simulink subsystem "luces"  (R2023b)
settings: Solver=VariableStepAuto  StartTime=0.0  StopTime=10.0  RelTol=1e-3
libraries: simulink x8
settings Model: Creator=Usuario_UMA  LastModifiedBy=fdcdm

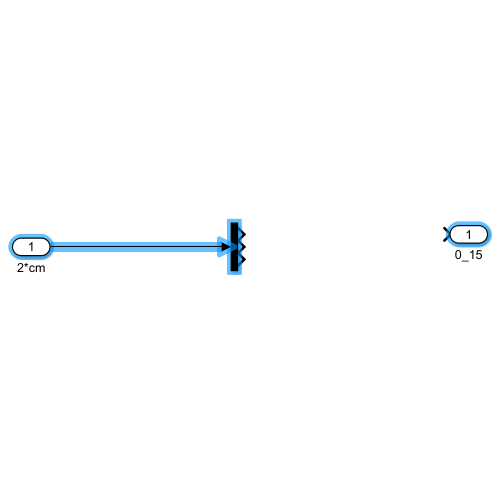
[thumbnail: Simulink's stored preview of the top-level diagram]
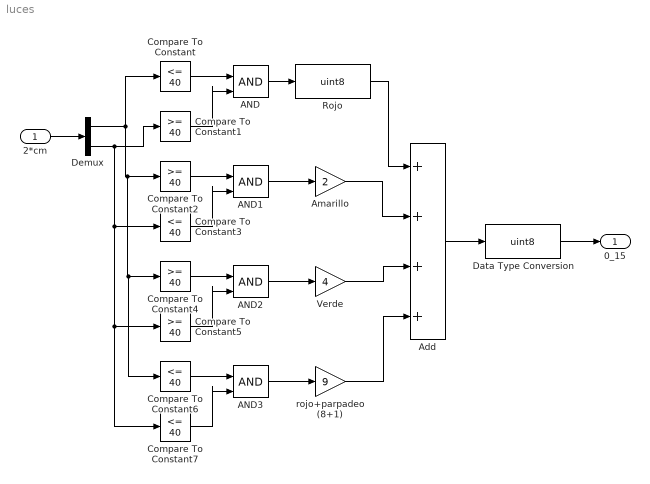
== system luces ==
  2*cm : Inport
  AND{,1..3} (4 alike) : Logic  IconShape=distinctive  AllPortsSameDT=off  OutDataTypeStr=boolean
  Add : Sum  Inputs=++++
  Amarillo : Gain  Gain=2
  Compare To Constant{,3,6..7} (4 alike) : simulink/Logic and Bit Operations/Compare To Constant  relop=<=  const=40  OutDataTypeStr=boolean
  Compare To Constant{1..2,4..5} (4 alike) : simulink/Logic and Bit Operations/Compare To Constant  relop=>=  const=40  OutDataTypeStr=boolean
  Data Type Conversion : DataTypeConversion  OutDataTypeStr=uint8  SaturateOnIntegerOverflow=off  RndMeth=Floor
  Demux : Demux  Outputs=2
  Rojo : DataTypeConversion  OutDataTypeStr=uint8  SaturateOnIntegerOverflow=off  RndMeth=Floor
  Verde : Gain  Gain=4
  rojo+parpadeo (8+1) : Gain  Gain=9
  0_15 : Outport  OutDataTypeStr=uint8
  wires:
  2*cm/1 -> Demux/1
  AND/1 -> Rojo/1
  Rojo/1 -> Add/1
  Compare To Constant/1 -> AND/1
  Compare To Constant1/1 -> AND/2
  Compare To Constant3/1 -> AND1/2
  Compare To Constant2/1 -> AND1/1
  Compare To Constant5/1 -> AND2/2
  Compare To Constant4/1 -> AND2/1
  AND2/1 -> Verde/1
  AND1/1 -> Amarillo/1
  Demux/2 -> Compare To Constant1/1, Compare To Constant3/1, Compare To Constant5/1, Compare To Constant7/1
  Compare To Constant7/1 -> AND3/2
  Demux/1 -> Compare To Constant/1, Compare To Constant2/1, Compare To Constant4/1, Compare To Constant6/1
  Compare To Constant6/1 -> AND3/1
  Amarillo/1 -> Add/2
  Verde/1 -> Add/3
  rojo+parpadeo (8+1)/1 -> Add/4
  AND3/1 -> rojo+parpadeo (8+1)/1
  Data Type Conversion/1 -> 0_15/1
  Add/1 -> Data Type Conversion/1
